simulink model "F4_CAN_LoopBackInterrupt"  (R2018b)
settings: Solver=FixedStepDiscrete  StartTime=0.0  StopTime=10.0  FixedStep=1  RelTol=1e-3  EnableMultiTasking=on
libraries: CAN_Lib x16, canmsglib x2, simulink x2, STM32_Config_Lib x1
settings Model: Creator=reynaudp  LastModifiedBy=fenard1
settings DataIOCC: LimitDataPoints=on  SaveFormat=Array
settings OptimizationCC: DefaultParameterBehavior=Inlined  DefaultUnderspecifiedDataType=single  PassReuseOutputArgsAs=Individual arguments  LifeSpan=1
settings DebuggingCC: ArrayBoundsChecking=error  SignalInfNanChecking=error  SolverPrmCheckMsg=warning  UniqueDataStoreMsg=error  AllowSymbolicDim=off  StrictBusMsg=ErrorOnBusTreatedAsVector  SFUnexpectedBacktrackingDiag=warning  SFNoUnconditionalDefaultTransitionDiag=warning  SFUndirectedBroadcastEventsDiag=error  SFExecutionAtInitializationDiag=none
settings HardwareCC: ProdBitPerPointer=32  ProdBitPerSizeT=32  ProdBitPerPtrDiffT=32  ProdLargestAtomicInteger=Integer  ProdWordSize=32  ProdHWDeviceType=STMicroelectronics->STM32 32-bit Cortex-M
settings ModelReferenceCC: PropagateSignalLabelsOutOfModel=off
settings SFSimCC: SimUseLocalCustomCode=off  CompileTimeRecursionLimit=0  EnableRuntimeRecursion=off  MATLABDynamicMemAlloc=off
settings RTWCC: SystemTargetFile=stm32.tlc  TemplateMakefile=stm32.tmf  Description=stm32 (Embedded Target)  GenerateReport=on  RTWVerbose=off  RTWUseLocalCustomCode=off  CustomDefine=RTWTYPES_H  Toolchain=Microsoft Windows SDK v7.1 | nmake (64-bit Windows)  IncludeHyperlinkInReport=on
settings CodeAppCC: IgnoreCustomStorageClasses=off  CustomSymbolStrType=$N$R$M  SimulinkBlockComments=off
settings STFCustomTargetCC: TargetLangStandard=C99 (ISO)  ParMdlRefBuildCompliant=on  IncludeMdlTerminateFcn=off  CombineOutputUpdateFcns=on  ERTCustomFileBanners=on  SupportComplex=off  SupportContinuousTime=off  SupportNonInlinedSFcns=off  RemoveResetFunc=on  ParenthesesLevel=Maximum  CastingMode=Standards  MATLABClassNameForMDSCustomization=Simulink.SoftwareTarget.ERTCustomization  SystemTargetFile=stm32.tlc
settings ERTTargetCC: TargetLangStandard=C99 (ISO)  MultiwordLength=2048  CompOptLevelCompliant=off  ConcurrentExecutionCompliant=off  IncludeMdlTerminateFcn=off  SupportComplex=off  ParenthesesLevel=Maximum  CastingMode=Standards  ModelStepFunctionPrototypeControlCompliant=off  CPPClassGenCompliant=off  UseToolchainInfoCompliant=off  ERTSrcFileBannerTemplate=sourceFileTemplate.cgt  ERTHdrFileBannerTemplate=sourceFileTemplate.cgt  ERTDataSrcFileTemplate=sourceFileTemplate.cgt  ERTDataHdrFileTemplate=sourceFileTemplate.cgt  ERTCustomFileTemplate=customRoutineProcess.tlc  ConvertIfToSwitch=off  SuppressUnreachableDefaultCases=off  EnableSignedLeftShifts=off  EnableSignedRightShifts=off
settings ConfigComp: CovMetricSettings=dw  CovHtmlReporting=on  CovSaveCumulativeToWorkspaceVar=on  CovSaveSingleToWorkspaceVar=on  CovExternalEMLEnable=off  CovSFcnEnable=off

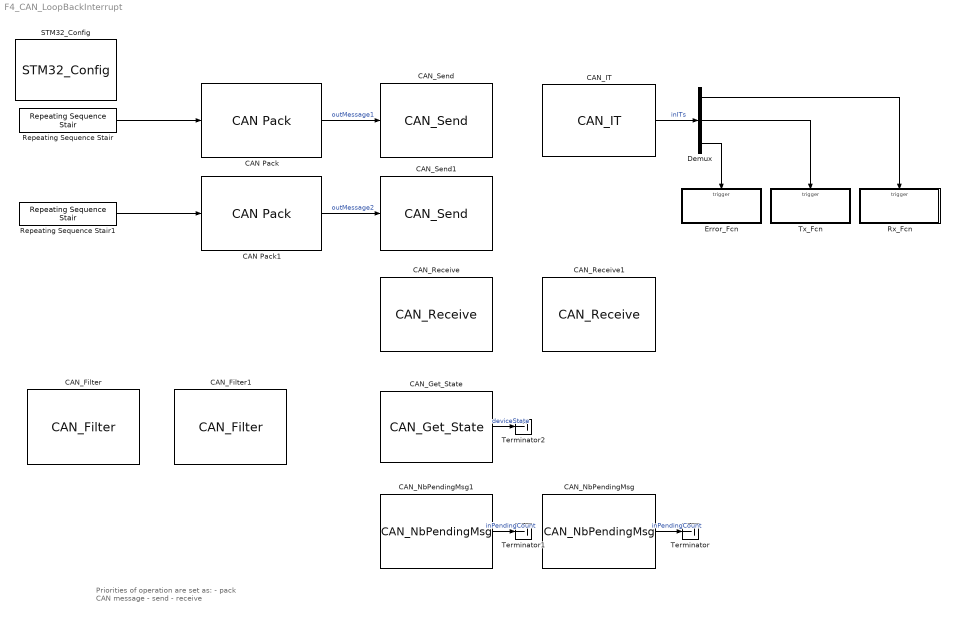
== system F4_CAN_LoopBackInterrupt ==
  note: Priorities of operation are set as:
      | - pack CAN message
      | - send
      | - receive
  CAN Pack : canmsglib/CAN Pack  Priority=1  MsgList=(none)  MsgName=CAN Msg  MsgIDType=Standard (11-bit identifier)  MsgIdentifier=100  MsgLength=8  SignalInfo=Signal1$0$8$1$1$1$0$1$0$-Inf$Inf$#  NSignals=1  StartBits=str2num('[int32(0)]')  SignalSizes=str2num('[int32(8)]')  ByteOrders=str2num('[int32(1)]')  DataTypes=str2num('[int32(1)]')  MultiplexTypes=str2num('[int32(1)]')  MultiplexValues=str2num('[double(0)]')  Factors=str2num('[double(1)]')  Offsets=str2num('[double(0)]')  Minimums=str2num('[double(-Inf)]')  Maximums=str2num('[double(Inf)]')  Remote=off  ApplyMinMax=off  BusOutput=off
      settings: AttributesFormatString=Priority=%<Priority>  SourceProductName=Simulink Real-Time  SourceProductBaseCode=XP  DataFormat=manually specified signals
  CAN Pack1 : canmsglib/CAN Pack  Priority=1  MsgList=(none)  MsgName=CAN Msg  MsgIDType=Standard (11-bit identifier)  MsgIdentifier=101  MsgLength=8  SignalInfo=Signal1$0$8$1$1$1$0$1$0$-Inf$Inf$#  NSignals=1  StartBits=str2num('[int32(0)]')  SignalSizes=str2num('[int32(8)]')  ByteOrders=str2num('[int32(1)]')  DataTypes=str2num('[int32(1)]')  MultiplexTypes=str2num('[int32(1)]')  MultiplexValues=str2num('[double(0)]')  Factors=str2num('[double(1)]')  Offsets=str2num('[double(0)]')  Minimums=str2num('[double(-Inf)]')  Maximums=str2num('[double(Inf)]')  Remote=off  ApplyMinMax=off  BusOutput=off
      settings: AttributesFormatString=Priority=%<Priority>  SourceProductName=Simulink Real-Time  SourceProductBaseCode=XP  DataFormat=manually specified signals
  CAN_Filter : CAN_Lib/CAN_Filter  CAN_name=CAN1  CAN_Filter_Activation=on  CAN_Filter_Scale=CAN_FILTERSCALE_32BIT  CAN_Filter_Mask_Id_High=65504  CAN_Filter_Mask_Id_Low=0  CAN_Filter_Id_High=3200  CAN_Filter_Id_Low=0  CAN_Filter_FIFO_Assignment=CAN_FIFO0  CAN_Filter_Bank=0  CAN_Filter_Mode=CAN_FILTERMODE_IDMASK  CAN_Filter_Slave_Start_Bank=14
      settings: SourceProductName=Target Support Package - STM32 Adapter
  CAN_Filter1 : CAN_Lib/CAN_Filter  CAN_name=CAN1  CAN_Filter_Activation=on  CAN_Filter_Scale=CAN_FILTERSCALE_16BIT  CAN_Filter_Mask_Id_High=65504  CAN_Filter_Mask_Id_Low=0  CAN_Filter_Id_High=3232  CAN_Filter_Id_Low=0  CAN_Filter_FIFO_Assignment=CAN_FIFO1  CAN_Filter_Bank=1  CAN_Filter_Mode=CAN_FILTERMODE_IDLIST  CAN_Filter_Slave_Start_Bank=14
      settings: SourceProductName=Target Support Package - STM32 Adapter
  CAN_Get_State : CAN_Lib/CAN_Get_State  CAN_name=CAN1
      settings: SourceProductName=Target Support Package - STM32 Adapter
  CAN_IT : CAN_Lib/CAN_IT  CAN_name=CAN1  CAN_Mode=Master  CAN_It=on  CAN_RX_It=on  CAN_TX_It=on  CAN_ERROR_It=on
      settings: SourceProductName=Target Support Package - STM32 Adapter
  CAN_NbPendingMsg : CAN_Lib/CAN_NbPendingMsg  CAN_name=CAN1  CAN_Mode=Master  CAN_It=on  CAN_Fifo=CAN_FIFO1
      settings: SourceProductName=Target Support Package - STM32 Adapter
  CAN_NbPendingMsg1 : CAN_Lib/CAN_NbPendingMsg  CAN_name=CAN1  CAN_Mode=Master  CAN_It=on  CAN_Fifo=CAN_FIFO0
      settings: SourceProductName=Target Support Package - STM32 Adapter
  CAN_Receive : CAN_Lib/CAN_Receive  Priority=3  CAN_name=CAN1  CAN_Mode=Master  CAN_It=on  CAN_Fifo=CAN_FIFO0
      settings: AttributesFormatString=Priority=%<Priority>  SourceProductName=Target Support Package - STM32 Adapter
  CAN_Receive1 : CAN_Lib/CAN_Receive  Priority=3  CAN_name=CAN1  CAN_Mode=Master  CAN_It=on  CAN_Fifo=CAN_FIFO1
      settings: AttributesFormatString=Priority=%<Priority>  SourceProductName=Target Support Package - STM32 Adapter
  CAN_Send : CAN_Lib/CAN_Send  Priority=2  CAN_name=CAN1  CAN_Mode=Master  CAN_It=on  CAN_MsgType=on
      settings: AttributesFormatString=Priority=%<Priority>  SourceProductName=Target Support Package - STM32 Adapter
  CAN_Send1 : CAN_Lib/CAN_Send  Priority=2  CAN_name=CAN1  CAN_Mode=Master  CAN_It=on  CAN_MsgType=on
      settings: AttributesFormatString=Priority=%<Priority>  SourceProductName=Target Support Package - STM32 Adapter
  Demux : Demux  Outputs=3
  Error_Fcn : Subsystem  TreatAsAtomicUnit=on
  Repeating Sequence Stair : simulink/Sources/Repeating Sequence Stair  OutValues=[1 2 3 4 5 6 7 8].'  tsamp=-1  OutMin=[]  OutMax=[]  OutDataTypeStr=uint8  OutputDataTypeScalingMode=uint8  OutDataType=fixdt(0,8)  ConRadixGroup=Best Precision: Vector-wise  OutScaling=2^-12
  Repeating Sequence Stair1 : simulink/Sources/Repeating Sequence Stair  OutValues=[11 12 13 14 15 16 17 18].'  tsamp=-1  OutMin=[]  OutMax=[]  OutDataTypeStr=uint8  OutputDataTypeScalingMode=uint8  OutDataType=fixdt(0,8)  ConRadixGroup=Best Precision: Vector-wise  OutScaling=2^-12
  Rx_Fcn : Subsystem  TreatAsAtomicUnit=on
  STM32_Config : STM32_Config_Lib/STM32_Config  Priority=0  Project_Path=.\  Config_File=F4_CAN_LoopBackInterrupt.ioc  MCU_Name=STM32F429ZITx
      settings: SourceProductName=Target Support Package - STM32 Adapter
  Terminator : Terminator
  Terminator1 : Terminator
  Terminator2 : Terminator
  Tx_Fcn : Subsystem  TreatAsAtomicUnit=on
  wires:
  CAN Pack/1 -> CAN_Send/1  "outMessage1"
  Repeating Sequence Stair/1 -> CAN Pack/1
  Demux/1 -> Rx_Fcn/Trigger
  Demux/2 -> Tx_Fcn/Trigger
  CAN_IT/1 -> Demux/1  "inITs"
  Demux/3 -> Error_Fcn/Trigger
  Repeating Sequence Stair1/1 -> CAN Pack1/1
  CAN Pack1/1 -> CAN_Send1/1  "outMessage2"
  CAN_NbPendingMsg/1 -> Terminator/1  "inPendingCount"
  CAN_NbPendingMsg1/1 -> Terminator1/1  "inPendingCount"
  CAN_Get_State/1 -> Terminator2/1  "deviceState"

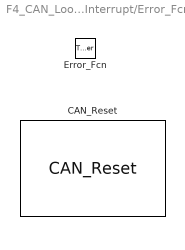
== system F4_CAN_LoopBackInterrupt/Error_Fcn ==
  Error_Fcn : TriggerPort  TriggerType=function-call  VariantControl=Variant
  CAN_Reset : CAN_Lib/CAN_Reset  CAN_name=CAN1
      settings: SourceProductName=Target Support Package - STM32 Adapter

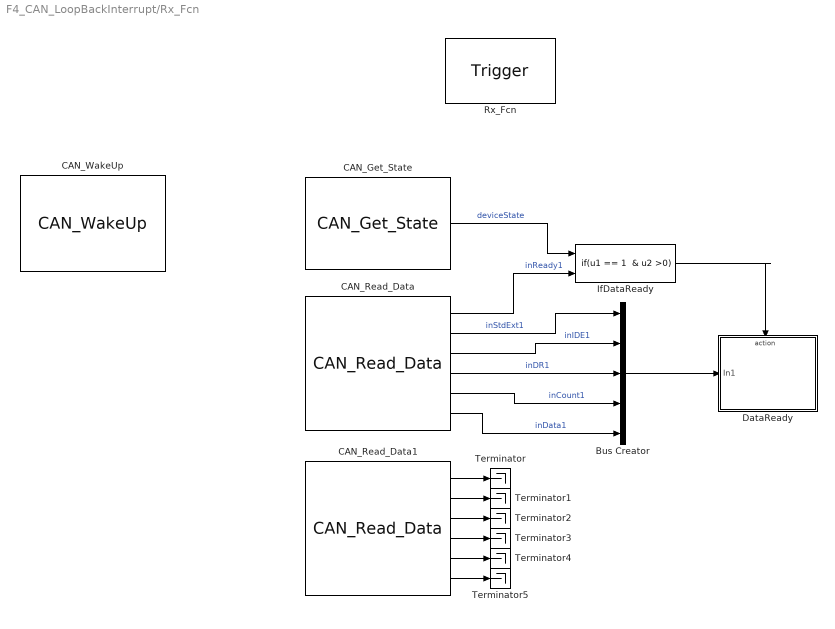
== system F4_CAN_LoopBackInterrupt/Rx_Fcn ==
  Rx_Fcn : TriggerPort  TriggerType=function-call  VariantControl=Variant
  Bus Creator : BusCreator  Inputs=5
  CAN_Get_State : CAN_Lib/CAN_Get_State  CAN_name=CAN1
      settings: SourceProductName=Target Support Package - STM32 Adapter
  CAN_Read_Data : CAN_Lib/CAN_Read_Data  CAN_name=CAN1  CAN_Fifo=CAN_FIFO0  CAN_MsgType=off
      settings: SourceProductName=Target Support Package - STM32 Adapter
  CAN_Read_Data1 : CAN_Lib/CAN_Read_Data  CAN_name=CAN1  CAN_Fifo=CAN_FIFO1  CAN_MsgType=off
      settings: SourceProductName=Target Support Package - STM32 Adapter
  CAN_WakeUp : CAN_Lib/CAN_WakeUp  CAN_name=CAN1  CAN_Mode=Master  CAN_It=on
      settings: SourceProductName=Target Support Package - STM32 Adapter
  DataReady : Subsystem  TreatAsAtomicUnit=on
  IfDataReady : If  NumInputs=2  IfExpression="u1 == 1  & u2 >0"  ShowElse=off
  Terminator{,1..5} (6 alike) : Terminator
  wires:
  CAN_Read_Data/6 -> Bus Creator/5  "inData1"
  CAN_Read_Data/5 -> Bus Creator/4  "inCount1"
  CAN_Read_Data/4 -> Bus Creator/3  "inDR1"
  CAN_Read_Data/1 -> IfDataReady/2  "inReady1"
  CAN_Read_Data/2 -> Bus Creator/1  "inStdExt1"
  CAN_Get_State/1 -> IfDataReady/1  "deviceState"
  Bus Creator/1 -> DataReady/1(In1)
  IfDataReady/1 -> DataReady/Action
  CAN_Read_Data/3 -> Bus Creator/2  "inIDE1"
  CAN_Read_Data1/1 -> Terminator/1
  CAN_Read_Data1/2 -> Terminator1/1
  CAN_Read_Data1/3 -> Terminator2/1
  CAN_Read_Data1/4 -> Terminator3/1
  CAN_Read_Data1/5 -> Terminator4/1
  CAN_Read_Data1/6 -> Terminator5/1

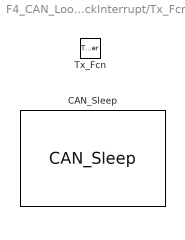
== system F4_CAN_LoopBackInterrupt/Tx_Fcn ==
  Tx_Fcn : TriggerPort  TriggerType=function-call  VariantControl=Variant
  CAN_Sleep : CAN_Lib/CAN_Sleep  CAN_name=CAN1  CAN_Mode=Master  CAN_It=on
      settings: SourceProductName=Target Support Package - STM32 Adapter

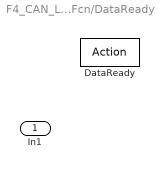
== system F4_CAN_LoopBackInterrupt/Rx_Fcn/DataReady ==
  In1 : Inport
  DataReady : ActionPort  ActionType=then
